simulink model "second"  (R2016b)
settings: Solver=VariableStepAuto  StartTime=0.0  StopTime=0.08  RelTol=1e-3
libraries: powerlib x31
settings Model: Creator=Youssef  LastModifiedBy=Youssef

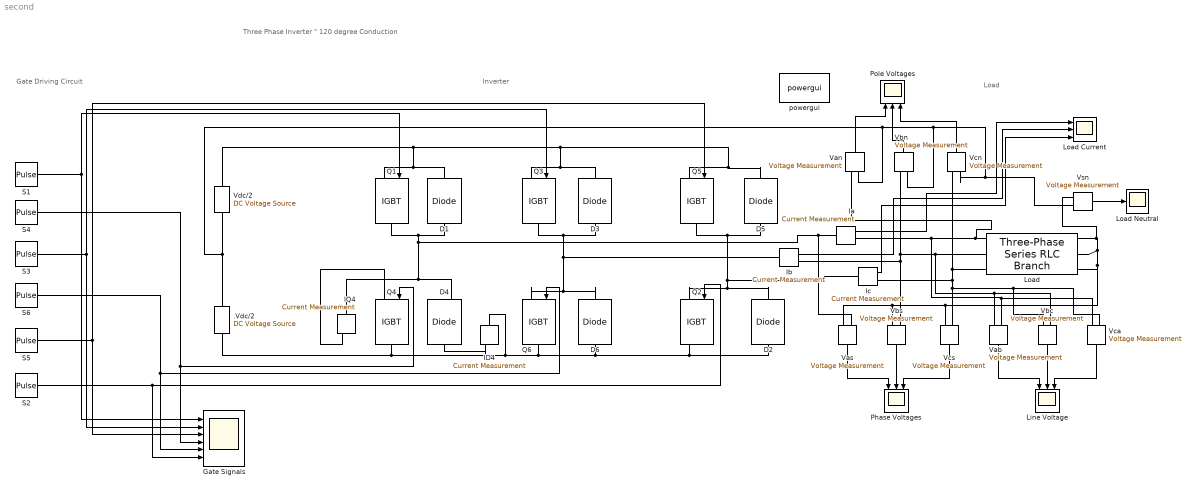
== system second ==
  note: Gate Driving Circuit
  note: Load
  note: Three Phase Inverter " 120 degree Conduction
  note: Inverter
  .Vdc/2 : powerlib/Electrical Sources/DC Voltage Source  Amplitude=100  Measurements=None
  D{1..3,5..6} (5 alike) : powerlib/Power Electronics/Diode  Ron=0.001  Lon=0  Vf=0.8  IC=0  UseSnubber=off  Rs=500  Cs=250e-9  Measurements=off
  D4 : powerlib/Power Electronics/Diode  Ron=0.001  Lon=0  Vf=0.8  IC=0  UseSnubber=off  Rs=500  Cs=250e-9  Measurements=on
  Gate Signals : Scope  NumInputPorts=6
  ID4 : powerlib/Measurements/Current Measurement  PhasorSimulation=off  OutputType=Complex  PSBequivalent=0
  IQ4 : powerlib/Measurements/Current Measurement  PhasorSimulation=off  OutputType=Complex  PSBequivalent=0
  Ia : powerlib/Measurements/Current Measurement  PhasorSimulation=off  OutputType=Complex  PSBequivalent=0
  Ib : powerlib/Measurements/Current Measurement  PhasorSimulation=off  OutputType=Complex  PSBequivalent=0
  Ic : powerlib/Measurements/Current Measurement  PhasorSimulation=off  OutputType=Complex  PSBequivalent=0
  Line Voltage : Scope  NumInputPorts=3
  Load : powerlib/Elements/Three-Phase Series RLC Branch  LConnTagsString=A|B|C  RConnTagsString=A|B|C  BranchType=R  Resistance=10  Inductance=1e-3  Capacitance=1e-6  Measurements=None
  Load Current : Scope  NumInputPorts=3
  Load Neutral : Scope
  Phase Voltages : Scope  NumInputPorts=3
  Pole Voltages : Scope  NumInputPorts=3
  Q{1,3..6} (5 alike) : powerlib/Power Electronics/IGBT  Ron=0.001  Lon=0  Vf=0.4  Tf=1e-6  Tt=2e-6  IC=0  Rs=1e5  Cs=inf  Measurements=off
  Q2 : powerlib/Power Electronics/IGBT  Ron=0.001  Lon=0  Vf=0.4  Tf=1e-6  Tt=2e-6  IC=0  Rs=1e5  Cs=inf  Measurements=on
  S1 : DiscretePulseGenerator  PulseType=Time based  Period=0.02  PulseWidth=100/3
  S2 : DiscretePulseGenerator  PulseType=Time based  Period=0.02  PulseWidth=100/3  PhaseDelay=(2*0.02/3)+(0.02/2)
  S3 : DiscretePulseGenerator  PulseType=Time based  Period=0.02  PulseWidth=100/3  PhaseDelay=0.02/3
  S4 : DiscretePulseGenerator  PulseType=Time based  Period=0.02  PulseWidth=100/3  PhaseDelay=0.02/2
  S5 : DiscretePulseGenerator  PulseType=Time based  Period=0.02  PulseWidth=100/3  PhaseDelay=(2*0.02)/3
  S6 : DiscretePulseGenerator  PulseType=Time based  Period=0.02  PulseWidth=100/3  PhaseDelay=(0.02/3)+(0.02/2)
  Vab : powerlib/Measurements/Voltage Measurement  PhasorSimulation=off  OutputType=Complex  PSBequivalent=0
  Van : powerlib/Measurements/Voltage Measurement  PhasorSimulation=off  OutputType=Complex  PSBequivalent=0
  Vas : powerlib/Measurements/Voltage Measurement  PhasorSimulation=off  OutputType=Complex  PSBequivalent=0
  Vbc : powerlib/Measurements/Voltage Measurement  PhasorSimulation=off  OutputType=Complex  PSBequivalent=0
  Vbn : powerlib/Measurements/Voltage Measurement  PhasorSimulation=off  OutputType=Complex  PSBequivalent=0
  Vbs : powerlib/Measurements/Voltage Measurement  PhasorSimulation=off  OutputType=Complex  PSBequivalent=0
  Vca : powerlib/Measurements/Voltage Measurement  PhasorSimulation=off  OutputType=Complex  PSBequivalent=0
  Vcn : powerlib/Measurements/Voltage Measurement  PhasorSimulation=off  OutputType=Complex  PSBequivalent=0
  Vcs : powerlib/Measurements/Voltage Measurement  PhasorSimulation=off  OutputType=Complex  PSBequivalent=0
  Vdc/2 : powerlib/Electrical Sources/DC Voltage Source  Amplitude=100  Measurements=None
  Vsn : powerlib/Measurements/Voltage Measurement  PhasorSimulation=off  OutputType=Complex  PSBequivalent=0
  powergui : powerlib/powergui  Priority=1  SimulationMode=Discrete  SolverType=Tustin/Backward Euler (TBE)  SampleTime=1e-6  frequency=60  SPID=off  DisableSnubberDevices=off  DisableRonSwitches=off  DisableVfSwitches=off  SwTol=0  DisplayEquations=off  Interpol=off  ExternalGateDelay=off  methode=off  Ts=10  FunctionMessages=off  echomessages=off  HookPort=off  EnableUseOfTLC=off  x0status=blocks  frequencyindice=0  Pbase=100e6  ErrMax=1e-4  Iterations=50  UnitsV=kV  UnitsW=MW  buscounter=0  RestoreLinks=warning  ResistiveCurrentMeasurement=off  Frange=[0:2:500]  Ylog=off  Xlog=on  ShowGrid=off  save=off  variable=ZData  structure=I  ZoomFFT=off  StartTime=0.02  cycles=2  DisplayStyle=1  fundamental=50  FreqAxis=off  MaxFrequency=1000  frequencyindicesteady=1  RmsSteady=1  display=off
  wires:
  S1/1 -> Gate Signals/1, Q1/1
  S3/1 -> Gate Signals/2, Q3/1
  S5/1 -> Q5/1, Gate Signals/3
  S6/1 -> Gate Signals/5, Q6/1
  Ia/1 -> Load Current/1
  Ib/1 -> Load Current/2
  Ic/1 -> Load Current/3
  Van/1 -> Pole Voltages/1
  Vbn/1 -> Pole Voltages/2
  Vcn/1 -> Pole Voltages/3
  Vas/1 -> Phase Voltages/1
  Vbs/1 -> Phase Voltages/2
  Vcs/1 -> Phase Voltages/3
  Vab/1 -> Line Voltage/1
  Vbc/1 -> Line Voltage/2
  Vca/1 -> Line Voltage/3
  Vsn/1 -> Load Neutral/1
  S4/1 -> Gate Signals/4, Q4/1
  S2/1 -> Gate Signals/6, Q2/1
  connections:
  Q1/LConn1 -- D1/RConn1 -- D5/RConn1 -- Q5/LConn1 -- Q3/LConn1 -- D3/RConn1 -- Vdc/2/RConn1
  D3/LConn1 -- Q3/RConn1 -- Ib/LConn1 -- D6/RConn1 -- Q6/LConn1
  Q5/RConn1 -- D5/LConn1 -- D2/RConn1 -- Q2/LConn1 -- Ic/LConn1
  .Vdc/2/RConn1 -- Vdc/2/LConn1 -- Vsn/LConn2 -- Vcn/LConn2 -- Vbn/LConn2 -- Van/LConn2
  Q4/RConn1 -- ID4/LConn1 -- D2/LConn1 -- Q2/RConn1 -- D6/LConn1 -- Q6/RConn1 -- .Vdc/2/LConn1
  Load/RConn2 -- Vas/LConn2 -- Vbs/LConn2 -- Vcs/LConn2 -- Load/RConn3 -- Load/RConn1 -- Vsn/LConn1
  Load/LConn1 -- Van/LConn1 -- Ia/RConn1 -- Vca/LConn2 -- Vab/LConn1
  Vbs/LConn1 -- Ib/RConn1 -- Vab/LConn2 -- Vbc/LConn1 -- Load/LConn2 -- Vbn/LConn1
  Load/LConn3 -- Vcn/LConn1 -- Ic/RConn1 -- Vca/LConn1 -- Vbc/LConn2 -- Vcs/LConn1
  D4/RConn1 -- Vas/LConn1 -- Ia/LConn1 -- Q1/RConn1 -- D1/LConn1 -- IQ4/LConn1
  IQ4/RConn1 -- Q4/LConn1
  ID4/RConn1 -- D4/LConn1
